simulink model "sm_flex_slider_crank"  (R2020b)
settings: Solver=ode23t  StartTime=0.0  StopTime=1.6  RelTol=1e-3  AbsTol=1e-3
PreLoadFcn:
  | if(~exist('shabanaCrankshaft','var'))
  |   load sliderCrankFEData
  | end
PostLoadFcn:
  | % Enable hard stop
  | hs_on = sm_flex_slider_crank_configure_hardstop(bdroot,'on');
undefined symbols (not defined in the file): beam_wall, beam_width, Extr_Data_Box, shabanaConnectingRod, shabanaCrankshaft, X, Y, Z
libraries: sm_lib x15, nesl_utility x7, sm_flex_body_lib x6, forcesPS_lib x1, fl_lib x1, simulink x1
CloseFcn:
  | try,close(h1_sm_flex_slider_crank),end
  | clear h1_sm_flex_slider_crank
  | try,close(h2_sm_flex_slider_crank),end
  | clear h2_sm_flex_slider_crank
  | try,close(h3_sm_flex_slider_crank),end
  | clear h3_sm_flex_slider_crank
  | try,close(h4_sm_flex_slider_crank),end
  | clear h4_sm_flex_slider_crank
  | 
  | 
  | clear simlog_sm_flex_slider_crank
  | clear logsout_sm_flex_slider_crank
Description:
  | Flexible Body Slider Crank
  | 
  | Copyright 2016-2020 The MathWorks, Inc.
settings Model: Creator=yvanwedd  LastModifiedBy=smiller
settings SolverCC: AutoScaleAbsTol=off
settings DataIOCC: MaxDataPoints=10000  ReturnWorkspaceOutputs=off  SignalLoggingName=logsout_sm_flex_slider_crank
settings DebuggingCC: PregeneratedLibrarySubsystemCodeDiagnostic=none  ArithmeticOperatorsInVariantConditions=warning
settings SFSimCC: SimUseLocalCustomCode=off  CustomCodeUndefinedFunction=UseInterfaceOnly
settings RTWCC: RTWUseLocalCustomCode=off
settings CodeAppCC: StateflowObjectComments=on
settings SimscapeCC: SimscapeNormalizeSystem=off  SimscapeLogType=all  SimscapeLogSimulationStatistics=on  SimscapeLogName=simlog_sm_flex_slider_crank  SimscapeLogLimitData=off  SimscapeLogDataHistory=10000
settings ExplorerConfigSet: InternalSimMechanicsExplorerSettings="<ExplorerConfiguration><canonicalview>default</canonicalview><AnimationSetting><BasePlaybackSpeed>1.0</BasePlaybackSpeed><PlaybackSpeedFactor>1.0</PlaybackSpeedFactor></AnimationSetting><TilePanel><TileInfo><Tiles Columns=\"1\" Count=\"1\" Rows=\"1\"><Column Left=\"2\" Weight=\"1\"/><Column Left=\"599\"/><Row Top=\"2\" Weight=\"1\"/><Row Top=\"397\"/><Tile Height=\"1\" Width=\"1\" X=\"0\" Y=\"0\"/></Tiles></TileInfo><SceneInfo><SceneViewer><BGColor><R>1</R><G>1</G><B>1</B></BGColor><Camera><DoPerspective>off</DoPerspective><Position><X>0.55203353364576724</X><Y>-0.22217409389501411</Y><Z>-0.85738767532460369</Z></Position><Center><X>0.16632771730262594</X><Y>-0.060781097290667566</Y><Z>0.051008341777047675</Z></Center><Up><X>-0.042698376474489097</X><Y>-0.98664868389108351</Y><Z>0.15716622799582453</Z></Up><ViewLimDist>1</ViewLimDist><YLim>0.19284836336170352</YLim><XLim>0.29376900947326862</XLim></Camera></SceneViewer></SceneInfo></TilePanel><MechEditorPanel><Cameras/><GfxPanelCameraMap/><VideoCreator><PlaybackSpeedRatio>1.0</PlaybackSpeedRatio><FrameRate>30</FrameRate><VideoFormat>Motion JPEG AVI</VideoFormat><FrameSize>auto</FrameSize></VideoCreator></MechEditorPanel></ExplorerConfiguration>"

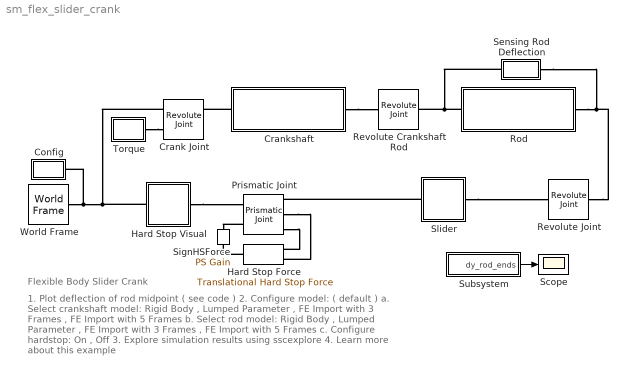
== system sm_flex_slider_crank ==
  note: Flexible Body Slider Crank
  note: 1. Plot deflection of rod midpoint ( see code )
      | 2. Configure model: ( default )
      | a. Select crankshaft model: Rigid Body , Lumped Parameter ,
      | FE Import with 3 Frames , FE Import with 5 Frames
      | b. Select rod model: Rigid Body , Lumped Parameter ,
      | FE Import with 3 Frames , FE Import with 5 Frames
      | c. Configure hardstop: On , Off
      | 3. Explore simulation results using sscexplore
      | 4. Learn more about this example
  Config : Subsystem
  Crank Joint : sm_lib/Joints/Revolute Joint  JointMode=Normal  SenseConstraintForce=off  SenseConstraintForceX=off  SenseConstraintForceY=off  SenseConstraintForceZ=off  SenseConstraintTorque=off  SenseConstraintTorqueX=off  SenseConstraintTorqueY=off  SenseConstraintTorqueZ=off  SenseTotalForce=off  SenseTotalForceX=off  SenseTotalForceY=off  SenseTotalForceZ=off  SenseTotalTorque=off  SenseTotalTorqueX=off  SenseTotalTorqueY=off  SenseTotalTorqueZ=off  CompositeWrenchDir=FollowerOnBase  CompositeWrenchFrame=BaseFrame  EquilibriumPosition=0  EquilibriumPositionUnits=deg  SpringStiffness=0  SpringStiffnessUnits=N*m/deg  DampingCoefficient=0  DampingCoefficientUnits=N*m/(deg/s)  TorqueActuationMode=InputTorque  MotionActuationMode=ComputedMotion  SensePosition=on  SenseVelocity=off  SenseAcceleration=off  SenseTorqueForce=off  SenseLowerLimitTorqueForce=off  SenseUpperLimitTorqueForce=off  LowerLimitSpecify=off  LowerLimitBound=-90  LowerLimitBoundUnits=deg  LowerLimitStiffness=1e4  LowerLimitStiffnessUnits=N*m/deg  LowerLimitDamping=10  LowerLimitDampingUnits=N*m/(deg/s)  LowerLimitTransitionRegionWidth=0.1  LowerLimitTransitionRegionWidthUnits=deg  UpperLimitSpecify=off  UpperLimitBound=90  UpperLimitBoundUnits=deg  UpperLimitStiffness=1e4  UpperLimitStiffnessUnits=N*m/deg  UpperLimitDamping=10  UpperLimitDampingUnits=N*m/(deg/s)  UpperLimitTransitionRegionWidth=0.1  UpperLimitTransitionRegionWidthUnits=deg  PositionTargetSpecify=off  PositionTargetPriority=High  PositionTargetValue=0  PositionTargetValueUnits=deg  VelocityTargetSpecify=off  VelocityTargetPriority=High  VelocityTargetValue=0  VelocityTargetValueUnits=deg/s
  Crankshaft : Subsystem  Variant=on  VariantControlMode=label  VariantControl=Variant1  LabelModeActiveChoice=Rigid_Body
      settings: AttributesFormatString=%<ActiveVariant>
      mask Display:
      | blk = find_system(gcbh, 'SearchDepth', 1, 'Parent', gcb, 'VariantObject', get_param(gcb,'activevariant'));
      | eval(get_param(blk, 'MaskDisplay'));
  Hard Stop Visual : Subsystem
      mask Display:
      | if(evalin('base','hs_on'))
      | patch([1 1 -1 -1],[0.5 1 1 0.5],[0.5 0.5 0.5]);
      | %patch([1 1 -1 -1],[-1 1 1 -1],[0.5 0.5 0.5]);
      | patch([1 1 -1 -1],-[0.5 1 1 0.5],[0.5 0.5 0.5]);
      | else
      | patch([1 1 -1 -1],[-1 1 1 -1],[1 1 1]);
      | end
      | 
      | plot(-2,-2)
      | plot(2,2)
  Hard Stop Force : forcesPS_lib/Mechanical/Translational Hard Stop Force  upper_bnd=0.5 m  lower_bnd=0.3 m  stiff_up=1e6 N/m  stiff_low=1e6 N/m  D_up=150 N/(m/s)  D_low=150 N/(m/s)
      settings: InternalSimscapePortConfiguration="{\"Bottom\":[],\"Left\":[{\"id\":\"v\",\"label\":\"v\",\"type\":\"input\"},{\"id\":\"p\",\"label\":\"p\",\"type\":\"input\"}],\"Right\":[{\"id\":\"f\",\"label\":\"f\",\"type\":\"output\"}],\"Top\":[]}"
  Prismatic Joint : sm_lib/Joints/Prismatic Joint  JointMode=Normal  SenseConstraintForce=off  SenseConstraintForceX=off  SenseConstraintForceY=off  SenseConstraintForceZ=off  SenseConstraintTorque=off  SenseConstraintTorqueX=off  SenseConstraintTorqueY=off  SenseConstraintTorqueZ=off  SenseTotalForce=off  SenseTotalForceX=off  SenseTotalForceY=off  SenseTotalForceZ=off  SenseTotalTorque=off  SenseTotalTorqueX=off  SenseTotalTorqueY=off  SenseTotalTorqueZ=off  CompositeWrenchDir=FollowerOnBase  CompositeWrenchFrame=BaseFrame  EquilibriumPosition=0  EquilibriumPositionUnits=m  SpringStiffness=0  SpringStiffnessUnits=N/m  DampingCoefficient=0  DampingCoefficientUnits=N/(m/s)  TorqueActuationMode=InputTorque  MotionActuationMode=ComputedMotion  SensePosition=on  SenseVelocity=on  SenseAcceleration=off  SenseTorqueForce=off  SenseLowerLimitTorqueForce=off  SenseUpperLimitTorqueForce=off  LowerLimitSpecify=off  LowerLimitBound=-1  LowerLimitBoundUnits=m  LowerLimitStiffness=1e6  LowerLimitStiffnessUnits=N/m  LowerLimitDamping=1e3  LowerLimitDampingUnits=N/(m/s)  LowerLimitTransitionRegionWidth=1e-4  LowerLimitTransitionRegionWidthUnits=m  UpperLimitSpecify=off  UpperLimitBound=1  UpperLimitBoundUnits=m  UpperLimitStiffness=1e6  UpperLimitStiffnessUnits=N/m  UpperLimitDamping=1e3  UpperLimitDampingUnits=N/(m/s)  UpperLimitTransitionRegionWidth=1e-4  UpperLimitTransitionRegionWidthUnits=m  PositionTargetSpecify=on  PositionTargetPriority=High  PositionTargetValue=shabanaCrankshaft.L+shabanaConnectingRod.L  PositionTargetValueUnits=m  VelocityTargetSpecify=on  VelocityTargetPriority=High  VelocityTargetValue=0  VelocityTargetValueUnits=m/s
  Revolute Crankshaft Rod : sm_lib/Joints/Revolute Joint  JointMode=Normal  SenseConstraintForce=off  SenseConstraintForceX=off  SenseConstraintForceY=off  SenseConstraintForceZ=off  SenseConstraintTorque=off  SenseConstraintTorqueX=off  SenseConstraintTorqueY=off  SenseConstraintTorqueZ=off  SenseTotalForce=off  SenseTotalForceX=off  SenseTotalForceY=off  SenseTotalForceZ=off  SenseTotalTorque=off  SenseTotalTorqueX=off  SenseTotalTorqueY=off  SenseTotalTorqueZ=off  CompositeWrenchDir=FollowerOnBase  CompositeWrenchFrame=BaseFrame  EquilibriumPosition=0  EquilibriumPositionUnits=deg  SpringStiffness=0  SpringStiffnessUnits=N*m/deg  DampingCoefficient=0  DampingCoefficientUnits=N*m/(deg/s)  TorqueActuationMode=NoTorque  MotionActuationMode=ComputedMotion  SensePosition=off  SenseVelocity=off  SenseAcceleration=off  SenseTorqueForce=off  SenseLowerLimitTorqueForce=off  SenseUpperLimitTorqueForce=off  LowerLimitSpecify=off  LowerLimitBound=-90  LowerLimitBoundUnits=deg  LowerLimitStiffness=1e4  LowerLimitStiffnessUnits=N*m/deg  LowerLimitDamping=10  LowerLimitDampingUnits=N*m/(deg/s)  LowerLimitTransitionRegionWidth=0.1  LowerLimitTransitionRegionWidthUnits=deg  UpperLimitSpecify=off  UpperLimitBound=90  UpperLimitBoundUnits=deg  UpperLimitStiffness=1e4  UpperLimitStiffnessUnits=N*m/deg  UpperLimitDamping=10  UpperLimitDampingUnits=N*m/(deg/s)  UpperLimitTransitionRegionWidth=0.1  UpperLimitTransitionRegionWidthUnits=deg  PositionTargetSpecify=off  PositionTargetPriority=High  PositionTargetValue=-180  PositionTargetValueUnits=deg  VelocityTargetSpecify=off  VelocityTargetPriority=High  VelocityTargetValue=0  VelocityTargetValueUnits=deg/s
  Revolute Joint : sm_lib/Joints/Revolute Joint  JointMode=Normal  SenseConstraintForce=off  SenseConstraintForceX=off  SenseConstraintForceY=off  SenseConstraintForceZ=off  SenseConstraintTorque=off  SenseConstraintTorqueX=off  SenseConstraintTorqueY=off  SenseConstraintTorqueZ=off  SenseTotalForce=off  SenseTotalForceX=off  SenseTotalForceY=off  SenseTotalForceZ=off  SenseTotalTorque=off  SenseTotalTorqueX=off  SenseTotalTorqueY=off  SenseTotalTorqueZ=off  CompositeWrenchDir=FollowerOnBase  CompositeWrenchFrame=BaseFrame  EquilibriumPosition=0  EquilibriumPositionUnits=deg  SpringStiffness=0  SpringStiffnessUnits=N*m/deg  DampingCoefficient=0  DampingCoefficientUnits=N*m/(deg/s)  TorqueActuationMode=NoTorque  MotionActuationMode=ComputedMotion  SensePosition=off  SenseVelocity=off  SenseAcceleration=off  SenseTorqueForce=off  SenseLowerLimitTorqueForce=off  SenseUpperLimitTorqueForce=off  LowerLimitSpecify=off  LowerLimitBound=-90  LowerLimitBoundUnits=deg  LowerLimitStiffness=1e4  LowerLimitStiffnessUnits=N*m/deg  LowerLimitDamping=10  LowerLimitDampingUnits=N*m/(deg/s)  LowerLimitTransitionRegionWidth=0.1  LowerLimitTransitionRegionWidthUnits=deg  UpperLimitSpecify=off  UpperLimitBound=90  UpperLimitBoundUnits=deg  UpperLimitStiffness=1e4  UpperLimitStiffnessUnits=N*m/deg  UpperLimitDamping=10  UpperLimitDampingUnits=N*m/(deg/s)  UpperLimitTransitionRegionWidth=0.1  UpperLimitTransitionRegionWidthUnits=deg  PositionTargetSpecify=off  PositionTargetPriority=High  PositionTargetValue=0  PositionTargetValueUnits=deg  VelocityTargetSpecify=off  VelocityTargetPriority=High  VelocityTargetValue=0  VelocityTargetValueUnits=deg/s
  Rod : Subsystem  Variant=on  VariantControlMode=label  VariantControl=Variant1  LabelModeActiveChoice=FE_Import_5Frames
      settings: AttributesFormatString=%<ActiveVariant>
      mask Display:
      | blk = find_system(gcbh, 'SearchDepth', 1, 'Parent', gcb, 'VariantObject', get_param(gcb,'activevariant'));
      | eval(get_param(blk, 'MaskDisplay'));
  Scope : Scope
  Sensing Rod Deflection : Subsystem
  SignHSForce : fl_lib/Physical Signals/Functions/PS Gain  Tag=on  gain=-hs_on
      settings: AttributesFormatString=%<Tag>
  Slider : Subsystem
      mask Display:
      | patch([1 1 -1 -1],[-1 1 1 -1],[0.5 0.5 0.5]);
      | plot(-2.5,-2.5)
      | plot(2.5,2.5)
  Subsystem : Subsystem
  Torque : Subsystem
      mask DialogControl Control2 Prompt: No Parameters
  World Frame : sm_lib/Frames and Transforms/World Frame
  wires:
  Subsystem/1(dy_rod_ends) -> Scope/1
  connections:
  Torque/RConn1 -- Crank Joint/LConn2
  Prismatic Joint/RConn2 -- Hard Stop Force/LConn2
  Prismatic Joint/RConn3 -- Hard Stop Force/LConn1
  Prismatic Joint/LConn2 -- SignHSForce/RConn1
  Crankshaft/LConn1 -- Crank Joint/RConn1
  Crankshaft/RConn1 -- Revolute Crankshaft Rod/LConn1
  Rod/LConn1 -- Sensing Rod Deflection/LConn1 -- Revolute Crankshaft Rod/RConn1
  Hard Stop Force/RConn1 -- SignHSForce/LConn1
  Revolute Joint/RConn1 -- Sensing Rod Deflection/RConn1 -- Rod/RConn1
  World Frame/RConn1 -- Hard Stop Visual/RConn1 -- Crank Joint/LConn1 -- Config/RConn1
  Hard Stop Visual/LConn1 -- Prismatic Joint/LConn1
  Slider/LConn1 -- Prismatic Joint/RConn1
  Slider/RConn1 -- Revolute Joint/LConn1

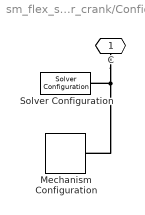
== system sm_flex_slider_crank/Config ==
  Mechanism Configuration : sm_lib/Utilities/Mechanism Configuration  UniformGravity=None  GravityVector=[0 0 -9.80665]  GravityVectorUnits=m/s^2  GravityUnits=m/s^2  LinearizationDelta=0.001  JointModeTransitionNonlinearIterations=2
  Solver Configuration : nesl_utility/Solver Configuration  PhysicalDomain=network_engine_domain  SubClassName=solver  LeftPortType=input  RightPortType=generic  Tones=[]  Harmonics=[]  SimulateNoise=off  Profile=off  UseLocalSampling=off  EnableSwitchedLinearOptims=on  FrequencyDomain=off  UseCCode=off  RelTol=0.001  AbsTol=1e-06  MinStep=1e-09  ToWorkspace=off  RevertToSquareIcSolve=off  NumHomotopyIterations=100  PhasorMode=off  PhasorModeNumHarmonics=1  DoDC=off  ResidualTolerance=1e-09  UseLocalSolver=off  LocalSolverChoice=NE_BACKWARD_EULER_ADVANCER  LocalSolverSampleTime=0.001  DoFixedCost=off  MaxNonlinIter=3  MaxModeIter=2  ComputeImpulses=off  ImpulseIterations=2  LinearAlgebra=Sparse  EquationFormulation=NE_TIME_EF  DelaysMemoryBudget=1024  AutomaticFiltering=on  FilteringTimeConstant=0.001  PartitionStorageMethod=AS_NEEDED  PartitionMemoryBudget=1024  PartitionMethod=FAST
  C : PMIOPort  Side=Right
  connections:
  Mechanism Configuration/RConn1 -- C/RConn1 -- Solver Configuration/RConn1

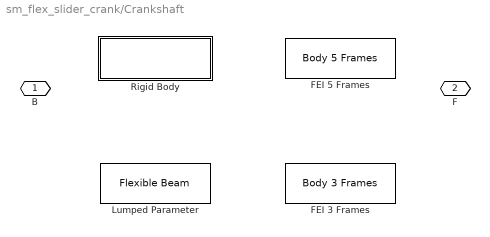
== system sm_flex_slider_crank/Crankshaft ==
  FEI 3 Frames : sm_flex_body_lib/FE Import/Bodies/Body 3 Frames  VariantControl=FE_Import_3Frames  popup_massdistr=Per Interface Frame  mass=shabanaCrankshaft.iner.mass  com=shabanaCrankshaft.iner.com  moi=shabanaCrankshaft.iner.moi  poi=shabanaCrankshaft.iner.poi  splitBodyProps=shabanaCrankshaft.splitBodyProps(2).props  smallInertiaDim=1e-2  smallInertiaMass=1e-4  rigid_body_filename='ShabanaCrankshaft.stl'  rigid_body_color=[0.5 0.5 0.5]  rigid_body_opacity=0  intf_body_color=[0.2 0.4 0.6]  intf_body_opacity=1  intf_graphic_color=[0.1 0.1 0.6]  intf_graphic_opacity=0  rigidBodyFrame=2  T=shabanaCrankshaft.models(5).T  numframes=3  K=shabanaCrankshaft.models(5).K  M=shabanaCrankshaft.models(5).M  ksi=0.05  dofIdxMap=shabanaCrankshaft.models(5).dofIdxMap  tau=1e-7  H=shabanaCrankshaft.models(5).H  sensedFeaDofs_UI=[]  numDynModes=20
      settings: AttributesFormatString=|
      | Mass: %<popup_massdistr>
      | Interface Frames: %<numframes>
      | Rigid Frame: %<rigidBodyFrame>
      | # Dynamic Modes: %<numDynModes>
  FEI 5 Frames : sm_flex_body_lib/FE Import/Bodies/Body 5 Frames  VariantControl=FE_Import_5Frames  popup_massdistr=Single  mass=shabanaCrankshaft.iner.mass  com=shabanaCrankshaft.iner.com  moi=shabanaCrankshaft.iner.moi  poi=shabanaCrankshaft.iner.poi  splitBodyProps=shabanaCrankshaft.splitBodyProps(3).props  smallInertiaDim=1e-2  smallInertiaMass=1e-4  rigid_body_filename='ShabanaCrankshaft.stl'  rigid_body_color=[0.5 0.5 0.5]  rigid_body_opacity=1  intf_body_color=[0.2 0.4 0.6]  intf_body_opacity=0  intf_graphic_color=[0.1 0.1 0.6]  intf_graphic_opacity=0  rigidBodyFrame=3  T=shabanaCrankshaft.models(7).T  numframes=5  K=shabanaCrankshaft.models(7).K  M=shabanaCrankshaft.models(7).M  ksi=0.05  dofIdxMap=shabanaCrankshaft.models(7).dofIdxMap  tau=1e-7  H=shabanaCrankshaft.models(7).H  sensedFeaDofs_UI=[]  numDynModes=20
      settings: AttributesFormatString=|
      | Mass: %<popup_massdistr>
      | Interface Frames: %<numframes>
      | Rigid Frame: %<rigidBodyFrame>
      | # Dynamic Modes: %<numDynModes>
  Lumped Parameter : sm_flex_body_lib/Lumped Parameter/Bodies/Flexible Beam  Tag=PublishSubsystem  VariantControl=Lumped_Parameter  popup_material=Custom  rho_cust=shabanaCrankshaft.mat.rho  youngsM_cust=shabanaCrankshaft.mat.E  shearM_cust=shabanaCrankshaft.mat.G  edf_beam=3.38e-05  sdf_beam=3.38e-05  checkbox_internalvalues=off  popup_xc=Hollow Rectangle  beam_width=shabanaCrankshaft.cs.b  beam_width_in=0  beam_height=shabanaCrankshaft.cs.a  beam_height_in=0  circle_diameter=0.015  circle_diameter_in=0  custom_ixx=2.6121e-003  custom_iyy=2.6121e-003  custom_ip=5.2242e-003  custom_j=5.2242e-003  extrusion_data_custom=[0.015 0.005;-0.015 0.005;-0.015 -0.005;0.015 -0.005]/2  beam_length=shabanaCrankshaft.L  elem_length=0.0152  numelem=10  extrusion_data=Extr_Data_Box(beam_width,beam_width-2*beam_wall,beam_width,beam_width-2*beam_wall)  beam_color=[0 0.4 0.6]  beam_opacity=1  radio_flextype=Rotation: Z
      settings: AttributesFormatString=|
      | No of Elem: 10
      | Rotation: Z
  Rigid Body : Subsystem  VariantControl=Rigid_Body
      mask Display: image('sm_flex_body_lib_rigidbody_IMAGE.png')
  " B " : PMIOPort  Side=Left
  " F " : PMIOPort  Port=2  Side=Right

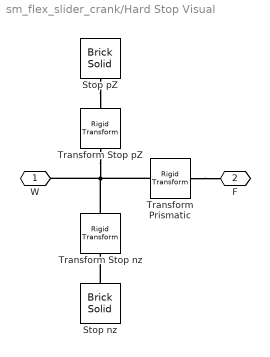
== system sm_flex_slider_crank/Hard Stop Visual ==
  Stop nz : sm_lib/Body Elements/Brick Solid  GraphicAmbientColor=[0.15 0.15 0.15 1.0]  BasedOnType=Density  BrickDimensions=[0.04 0.02 0.02]  BrickDimensionUnits=m  CenterOfMass=[0 0 0]  CenterOfMassUnits=m  GraphicDiffuseColor=[0.5 0.5 0.5]  Density=1000  DensityUnits=kg/m^3  DoExposeReferenceFrame=off  GraphicEmissiveColor=[0.0 0.0 0.0 1.0]  ExportEntireGeometry=off  SerializedFrames=<Frames><Frame><Id>Frame1</Id><Value><Name>F</Name><Origin><Source>GeometricFeature</Source><FeatureName>-z +x curve</FeatureName></Origin><PrimaryAxis><DefinedDirection>+Z</DefinedDirection><Source>ReferenceFrame</Source><SourceDirection>+Z</SourceDirection><FeatureName></FeatureName></PrimaryAxis><SecondaryAxis><DefinedDirection>+Y</DefinedDirection><Source>ReferenceFrame</Source><SourceDirection>+Y</SourceDirection><FeatureName></FeatureName></SecondaryAxis></Value></Frame></Frames>  MarkerShape=Sphere  MarkerSize=10  GraphicType=FromGeometry  InertiaType=PointMass  Mass=0  MassUnits=kg  MomentsOfInertia=[1 1 1]  MomentsOfInertiaUnits=kg*m^2  GraphicOpacity=hs_on*0.5  ProductsOfInertia=[1 1 1]  ProductsOfInertiaUnits=kg*m^2  GraphicShininess=75  GraphicSpecularColor=[0.5 0.5 0.5 1.0]  GraphicVisPropType=SimpleVisualProperties
  Stop pZ : sm_lib/Body Elements/Brick Solid  GraphicAmbientColor=[0.15 0.15 0.15 1.0]  BasedOnType=Density  BrickDimensions=[0.04 0.02 0.02]  BrickDimensionUnits=m  CenterOfMass=[0 0 0]  CenterOfMassUnits=m  GraphicDiffuseColor=[0.5 0.5 0.5]  Density=1000  DensityUnits=kg/m^3  DoExposeReferenceFrame=off  GraphicEmissiveColor=[0.0 0.0 0.0 1.0]  ExportEntireGeometry=off  SerializedFrames=<Frames><Frame><Id>Frame1</Id><Value><Name>F</Name><Origin><Source>GeometricFeature</Source><FeatureName>+z +x curve</FeatureName></Origin><PrimaryAxis><DefinedDirection>+Z</DefinedDirection><Source>ReferenceFrame</Source><SourceDirection>+Z</SourceDirection><FeatureName></FeatureName></PrimaryAxis><SecondaryAxis><DefinedDirection>+Y</DefinedDirection><Source>ReferenceFrame</Source><SourceDirection>+Y</SourceDirection><FeatureName></FeatureName></SecondaryAxis></Value></Frame></Frames>  MarkerShape=Sphere  MarkerSize=10  GraphicType=FromGeometry  InertiaType=PointMass  Mass=0  MassUnits=kg  MomentsOfInertia=[1 1 1]  MomentsOfInertiaUnits=kg*m^2  GraphicOpacity=hs_on*0.5  ProductsOfInertia=[1 1 1]  ProductsOfInertiaUnits=kg*m^2  GraphicShininess=75  GraphicSpecularColor=[0.5 0.5 0.5 1.0]  GraphicVisPropType=SimpleVisualProperties
  Transform Prismatic : sm_lib/Frames and Transforms/Rigid Transform  TranslationMethod=None  TranslationStandardOffset=0  TranslationLengthUnit=m  TranslationStandardAxis=+Z  TranslationCartesianOffset=[0 0 0]  TranslationROffset=0  TranslationROffsetUnits=m  TranslationZOffset=0  TranslationZOffsetUnits=m  TranslationThetaOffset=0  TranslationThetaOffsetUnits=deg  RotationMethod=StandardAxis  RotationAngleUnits=deg  RotationStandardAxis=+Y  RotationAngle=90  RotationArbitraryAxis=[0 0 1]  FollAlignAxisA=+X  BaseAlignAxisA=+Y  FollAlignAxisB=+Y  BaseAlignAxisB=+Z  RotationSequenceAxes=FollowerAxes  RotationSequence=XYX  RotationSequenceAngles=[0 0 0]  RotationSequenceAnglesUnits=deg  RotationMatrix=[1 0 0; 0 1 0; 0 0 1]
  Transform Stop nz : sm_lib/Frames and Transforms/Rigid Transform  TranslationMethod=Cartesian  TranslationStandardOffset=0  TranslationLengthUnit=m  TranslationStandardAxis=-Z  TranslationCartesianOffset=[0.3 0 shabanaConnectingRod.cs.a]  TranslationROffset=0  TranslationROffsetUnits=m  TranslationZOffset=0  TranslationZOffsetUnits=m  TranslationThetaOffset=0  TranslationThetaOffsetUnits=deg  RotationMethod=None  RotationAngleUnits=deg  RotationStandardAxis=+Y  RotationAngle=90  RotationArbitraryAxis=[0 0 1]  FollAlignAxisA=+X  BaseAlignAxisA=+Y  FollAlignAxisB=+Y  BaseAlignAxisB=+Z  RotationSequenceAxes=FollowerAxes  RotationSequence=XYX  RotationSequenceAngles=[0 0 0]  RotationSequenceAnglesUnits=deg  RotationMatrix=[1 0 0; 0 1 0; 0 0 1]
  Transform Stop pZ : sm_lib/Frames and Transforms/Rigid Transform  TranslationMethod=Cartesian  TranslationStandardOffset=0  TranslationLengthUnit=m  TranslationStandardAxis=-Z  TranslationCartesianOffset=[0.3 0 -shabanaConnectingRod.cs.a]  TranslationROffset=0  TranslationROffsetUnits=m  TranslationZOffset=0  TranslationZOffsetUnits=m  TranslationThetaOffset=0  TranslationThetaOffsetUnits=deg  RotationMethod=None  RotationAngleUnits=deg  RotationStandardAxis=+Y  RotationAngle=90  RotationArbitraryAxis=[0 0 1]  FollAlignAxisA=+X  BaseAlignAxisA=+Y  FollAlignAxisB=+Y  BaseAlignAxisB=+Z  RotationSequenceAxes=FollowerAxes  RotationSequence=XYX  RotationSequenceAngles=[0 0 0]  RotationSequenceAnglesUnits=deg  RotationMatrix=[1 0 0; 0 1 0; 0 0 1]
  W : PMIOPort  Side=Right
  F : PMIOPort  Port=2  Side=Left
  connections:
  Transform Prismatic/LConn1 -- Transform Stop nz/LConn1 -- Transform Stop pZ/LConn1 -- W/RConn1
  Transform Prismatic/RConn1 -- F/RConn1
  Stop pZ/LConn1 -- Transform Stop pZ/RConn1
  Stop nz/LConn1 -- Transform Stop nz/RConn1

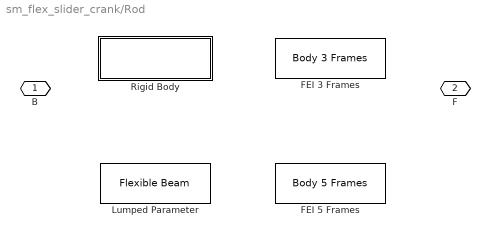
== system sm_flex_slider_crank/Rod ==
  FEI 3 Frames : sm_flex_body_lib/FE Import/Bodies/Body 3 Frames  VariantControl=FE_Import_3Frames  popup_massdistr=Per Interface Frame  mass=shabanaConnectingRod.iner.mass  com=shabanaConnectingRod.iner.com  moi=shabanaConnectingRod.iner.moi  poi=shabanaConnectingRod.iner.poi  splitBodyProps=shabanaConnectingRod.splitBodyProps(2).props  smallInertiaDim=1e-3  smallInertiaMass=1e-6  rigid_body_filename='ShabanaConnectingRod.step'  rigid_body_color=[0.5 0.5 0.5]  rigid_body_opacity=0  intf_body_color=[0.2 0.4 0.6]  intf_body_opacity=1  intf_graphic_color=[0.1 0.1 0.6]  intf_graphic_opacity=0  rigidBodyFrame=2  T=shabanaConnectingRod.models(5).T  numframes=3  K=shabanaConnectingRod.models(5).K  M=shabanaConnectingRod.models(5).M  ksi=0.05  dofIdxMap=shabanaConnectingRod.models(5).dofIdxMap  tau=1e-7  H=shabanaConnectingRod.models(5).H  sensedFeaDofs_UI=[]  numDynModes=20
      settings: AttributesFormatString=|
      | Mass: %<popup_massdistr>
      | Interface Frames: %<numframes>
      | Rigid Frame: %<rigidBodyFrame>
      | # Dynamic Modes: %<numDynModes>
  FEI 5 Frames : sm_flex_body_lib/FE Import/Bodies/Body 5 Frames  VariantControl=FE_Import_5Frames  popup_massdistr=Per Interface Frame  mass=shabanaConnectingRod.iner.mass  com=shabanaConnectingRod.iner.com  moi=shabanaConnectingRod.iner.moi  poi=shabanaConnectingRod.iner.poi  splitBodyProps=shabanaConnectingRod.splitBodyProps(3).props  smallInertiaDim=1e-3  smallInertiaMass=1e-6  rigid_body_filename='ShabanaConnectingRod.stl'  rigid_body_color=[0.5 0.5 0.5]  rigid_body_opacity=0  intf_body_color=[0.2 0.4 0.6]  intf_body_opacity=1  intf_graphic_color=[0.1 0.1 0.6]  intf_graphic_opacity=0  rigidBodyFrame=3  T=shabanaConnectingRod.models(7).T  numframes=5  K=shabanaConnectingRod.models(7).K  M=shabanaConnectingRod.models(7).M  ksi=0.05  dofIdxMap=shabanaConnectingRod.models(7).dofIdxMap  tau=1e-7  H=shabanaConnectingRod.models(7).H  sensedFeaDofs_UI=[]  numDynModes=20
      settings: AttributesFormatString=|
      | Mass: %<popup_massdistr>
      | Interface Frames: %<numframes>
      | Rigid Frame: %<rigidBodyFrame>
      | # Dynamic Modes: %<numDynModes>
  Lumped Parameter : sm_flex_body_lib/Lumped Parameter/Bodies/Flexible Beam  Tag=PublishSubsystem  VariantControl=Lumped_Parameter  popup_material=Custom  rho_cust=shabanaConnectingRod.mat.rho  youngsM_cust=shabanaConnectingRod.mat.E  shearM_cust=shabanaConnectingRod.mat.G  edf_beam=6.03e-04  sdf_beam=6.03e-04  checkbox_internalvalues=off  popup_xc=Hollow Rectangle  beam_width=shabanaConnectingRod.cs.b  beam_width_in=0  beam_height=shabanaConnectingRod.cs.a  beam_height_in=0  circle_diameter=0.015  circle_diameter_in=0  custom_ixx=2.6121e-003  custom_iyy=2.6121e-003  custom_ip=5.2242e-003  custom_j=5.2242e-003  extrusion_data_custom=[0.015 0.005;-0.015 0.005;-0.015 -0.005;0.015 -0.005]/2  beam_length=shabanaConnectingRod.L  elem_length=0.0152  numelem=20  extrusion_data=Extr_Data_Box(beam_width,beam_width-2*beam_wall,beam_width,beam_width-2*beam_wall)  beam_color=[0.6 0.4 0]  beam_opacity=1  radio_flextype=Rotation: Z
      settings: AttributesFormatString=|
      | No of Elem: 20
      | Rotation: Z
  Rigid Body : Subsystem  VariantControl=Rigid_Body
      mask Display: image('sm_flex_body_lib_rigidbody_IMAGE.png')
  " B " : PMIOPort  Side=Left
  " F " : PMIOPort  Port=2  Side=Right

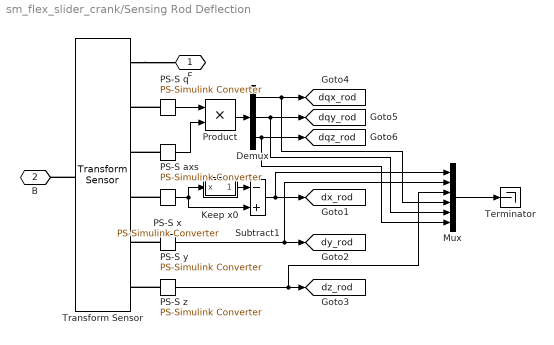
== system sm_flex_slider_crank/Sensing Rod Deflection ==
  Demux : Demux  Outputs=3
  Keep x0 : Subsystem
  Mux : Mux  Inputs=6
  PS-S axs : nesl_utility/PS-Simulink Converter  PhysicalDomain=network_engine_domain  SubClassName=ps_output  LeftPortType=input  RightPortType=output  PseudoPeriodic=off  Frequencies=[]  Unit=1  AffineConversion=off
  PS-S q : nesl_utility/PS-Simulink Converter  PhysicalDomain=network_engine_domain  SubClassName=ps_output  LeftPortType=input  RightPortType=output  PseudoPeriodic=off  Frequencies=[]  Unit=rad  AffineConversion=off
  PS-S x : nesl_utility/PS-Simulink Converter  PhysicalDomain=network_engine_domain  SubClassName=ps_output  LeftPortType=input  RightPortType=output  PseudoPeriodic=off  Frequencies=[]  Unit=m  AffineConversion=off
  PS-S y : nesl_utility/PS-Simulink Converter  PhysicalDomain=network_engine_domain  SubClassName=ps_output  LeftPortType=input  RightPortType=output  PseudoPeriodic=off  Frequencies=[]  Unit=m  AffineConversion=off
  PS-S z : nesl_utility/PS-Simulink Converter  PhysicalDomain=network_engine_domain  SubClassName=ps_output  LeftPortType=input  RightPortType=output  PseudoPeriodic=off  Frequencies=[]  Unit=m  AffineConversion=off
  Product : Product
  Subtract1 : Sum  Inputs=-+
  Terminator : Terminator
  Transform Sensor : sm_lib/Frames and Transforms/Transform Sensor  MeasurementFrame=Base  SenseAngle=on  SenseAxis=on  SenseAngle1=off  SenseAngle2=off  SenseAngle3=off  SenseQ=off  SenseR=off  SenseOmegaX=off  SenseOmegaY=off  SenseOmegaZ=off  SenseOmega1=off  SenseOmega2=off  SenseOmega3=off  SenseQDot=off  SenseRDot=off  SenseAlphaX=off  SenseAlphaY=off  SenseAlphaZ=off  SenseAlpha1=off  SenseAlpha2=off  SenseAlpha3=off  SenseQDDot=off  SenseRDDot=off  SenseX=on  SenseY=on  SenseZ=on  SenseRad=off  SenseAzim=off  SenseDist=off  SenseInc=off  SenseXDot=off  SenseYDot=off  SenseZDot=off  SenseRadDot=off  SenseAzimDot=off  SenseDistDot=off  SenseIncDot=off  SenseXDDot=off  SenseYDDot=off  SenseZDDot=off  SenseRadDDot=off  SenseAzimDDot=off  SenseDistDDot=off  SenseIncDDot=off
  F : PMIOPort  Side=Right
  B : PMIOPort  Port=2  Side=Left
  tag scope: dqx_rod=global, dqy_rod=global, dqz_rod=global, dx_rod=global, dy_rod=global, dz_rod=global
  wires:
  PS-S axs/1 -> Product/2
  PS-S q/1 -> Product/1
  PS-S z/1 -> Mux/3, [dz_rod]
  PS-S y/1 -> Mux/2, [dy_rod]
  Mux/1 -> Terminator/1
  Product/1 -> Demux/1
  Demux/1 -> Mux/4, [dqx_rod]
  Demux/2 -> [dqy_rod], Mux/5
  Demux/3 -> Mux/6, [dqz_rod]
  Subtract1/1 -> [dx_rod], Mux/1
  PS-S x/1 -> Keep x0/1(x), Subtract1/2
  Keep x0/1(x0) -> Subtract1/1
  connections:
  PS-S y/LConn1 -- Transform Sensor/RConn5
  PS-S axs/LConn1 -- Transform Sensor/RConn3
  Transform Sensor/RConn1 -- F/RConn1
  PS-S q/LConn1 -- Transform Sensor/RConn2
  Transform Sensor/LConn1 -- B/RConn1
  PS-S x/LConn1 -- Transform Sensor/RConn4
  PS-S z/LConn1 -- Transform Sensor/RConn6

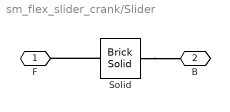
== system sm_flex_slider_crank/Slider ==
  Solid : sm_lib/Body Elements/Brick Solid  GraphicAmbientColor=[0.15 0.15 0.15 1.0]  BasedOnType=Density  BrickDimensions=[0.04 0.02 0.04]  BrickDimensionUnits=m  CenterOfMass=[0 0 0]  CenterOfMassUnits=m  GraphicDiffuseColor=[0.5 0.5 0.5]  Density=1000  DensityUnits=kg/m^3  DoExposeReferenceFrame=off  GraphicEmissiveColor=[0.0 0.0 0.0 1.0]  ExportEntireGeometry=off  SerializedFrames=<Frames><Frame><Id>Frame1</Id><Value><Name>F</Name><Origin><Source>GeometricFeature</Source><FeatureName>-x surface</FeatureName></Origin><PrimaryAxis><DefinedDirection>+Z</DefinedDirection><Source>ReferenceFrame</Source><SourceDirection>+X</SourceDirection><FeatureName></FeatureName></PrimaryAxis><SecondaryAxis><DefinedDirection>+Y</DefinedDirection><Source>ReferenceFrame</Source><SourceDirection>+Y</SourceDirection><FeatureName></FeatureName></SecondaryAxis></Value></Frame><Frame><Id>Frame2</Id><Value><Name>B</Name><Origin><Source>GeometricFeature</Source><FeatureName>-x surface</FeatureName></Origin><PrimaryAxis><DefinedDirection>+Z</DefinedDirection><Source>ReferenceFrame</Source><SourceDirection>+Z</SourceDirection><FeatureName></FeatureName></PrimaryAxis><SecondaryAxis><DefinedDirection>+X</DefinedDirection><Source>ReferenceFrame</Source><SourceDirection>+X</SourceDirection><FeatureName></FeatureName></SecondaryAxis></Value></Frame></Frames>  MarkerShape=Sphere  MarkerSize=10  GraphicType=FromGeometry  InertiaType=PointMass  Mass=0  MassUnits=kg  MomentsOfInertia=[1 1 1]  MomentsOfInertiaUnits=kg*m^2  GraphicOpacity=0.5  ProductsOfInertia=[1 1 1]  ProductsOfInertiaUnits=kg*m^2  GraphicShininess=75  GraphicSpecularColor=[0.5 0.5 0.5 1.0]  GraphicVisPropType=SimpleVisualProperties
  F : PMIOPort  Side=Left
  B : PMIOPort  Port=2  Side=Right
  connections:
  Solid/RConn1 -- B/RConn1
  Solid/LConn1 -- F/RConn1

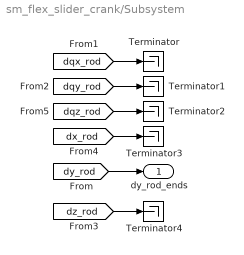
== system sm_flex_slider_crank/Subsystem ==
  Terminator{,1..4} (5 alike) : Terminator
  dy_rod_ends : Outport  VectorParamsAs1DForOutWhenUnconnected=off
  wires:
  [dy_rod] -> dy_rod_ends/1
  [dqx_rod] -> Terminator/1
  [dqy_rod] -> Terminator1/1
  [dqz_rod] -> Terminator2/1
  [dx_rod] -> Terminator3/1
  [dz_rod] -> Terminator4/1

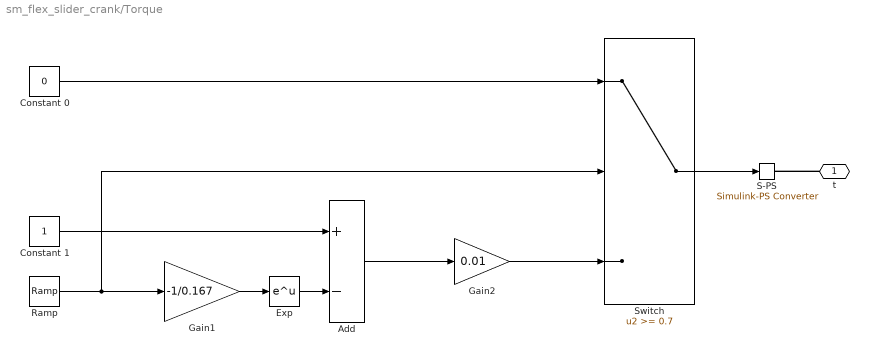
== system sm_flex_slider_crank/Torque ==
  Add : Sum  Inputs=+-
  Constant 0 : Constant  Value=0
  Constant 1 : Constant
  Exp : Math  SignedPower=on  SaturateOnIntegerOverflow=on
  Gain1 : Gain  Gain=-1/0.167
  Gain2 : Gain  Gain=0.01
  Ramp : simulink/Sources/Ramp  slope=1  start=0  InitialOutput=0
  S-PS : nesl_utility/Simulink-PS Converter  PhysicalDomain=network_engine_domain  SubClassName=ps_input  LeftPortType=input  RightPortType=output  PseudoPeriodic=off  Frequencies=[]  NoiseDistribution=none  NoiseParameters=[]  Unit=N*m  AffineConversion=off  FilteringAndDerivatives=zero  SimscapeFilterOrder=1  InputFilterTimeConstant=0.001  UdotUserProvided=1
  Switch : Switch  Threshold=0.7
  t : PMIOPort  Side=Right
  wires:
  Switch/1 -> S-PS/1
  Gain2/1 -> Switch/3
  Constant 0/1 -> Switch/1
  Exp/1 -> Add/2
  Constant 1/1 -> Add/1
  Add/1 -> Gain2/1
  Gain1/1 -> Exp/1
  Ramp/1 -> Gain1/1, Switch/2
  connections:
  t/RConn1 -- S-PS/RConn1

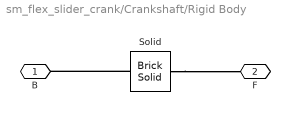
== system sm_flex_slider_crank/Crankshaft/Rigid Body ==
  Solid : sm_lib/Body Elements/Brick Solid  GraphicAmbientColor=[0.15 0.15 0.15 1.0]  BasedOnType=Density  BrickDimensions=[shabanaCrankshaft.L shabanaCrankshaft.cs.b shabanaCrankshaft.cs.a]  BrickDimensionUnits=m  CenterOfMass=[0 0 0]  CenterOfMassUnits=m  GraphicDiffuseColor=[0.5 0.5 0.5]  Density=1000  DensityUnits=kg/m^3  DoExposeReferenceFrame=off  GraphicEmissiveColor=[0.0 0.0 0.0 1.0]  ExportEntireGeometry=off  SerializedFrames=<Frames><Frame><Id>Frame1</Id><Value><Name>B</Name><Origin><Source>GeometricFeature</Source><FeatureName>-x surface</FeatureName></Origin><PrimaryAxis><DefinedDirection>+Z</DefinedDirection><Source>ReferenceFrame</Source><SourceDirection>+Z</SourceDirection><FeatureName></FeatureName></PrimaryAxis><SecondaryAxis><DefinedDirection>+X</DefinedDirection><Source>ReferenceFrame</Source><SourceDirection>+X</SourceDirection><FeatureName></FeatureName></SecondaryAxis></Value></Frame><Frame><Id>Frame2</Id><Value><Name>F</Name><Origin><Source>GeometricFeature</Source><FeatureName>+x surface</FeatureName></Origin><PrimaryAxis><DefinedDirection>+Z</DefinedDirection><Source>ReferenceFrame</Source><SourceDirection>+Z</SourceDirection><FeatureName></FeatureName></PrimaryAxis><SecondaryAxis><DefinedDirection>+X</DefinedDirection><Source>ReferenceFrame</Source><SourceDirection>+X</SourceDirection><FeatureName></FeatureName></SecondaryAxis></Value></Frame></Frames>  MarkerShape=Sphere  MarkerSize=10  GraphicType=FromGeometry  InertiaType=Custom  Mass=shabanaCrankshaft.iner.mass  MassUnits=kg  MomentsOfInertia=shabanaCrankshaft.iner.moi  MomentsOfInertiaUnits=kg*m^2  GraphicOpacity=1.0  ProductsOfInertia=shabanaCrankshaft.iner.poi  ProductsOfInertiaUnits=kg*m^2  GraphicShininess=75  GraphicSpecularColor=[0.5 0.5 0.5 1.0]  GraphicVisPropType=SimpleVisualProperties
  " B " : PMIOPort  Side=Left
  " F " : PMIOPort  Port=2  Side=Right
  connections:
  Solid/LConn1 -- " B "/RConn1
  Solid/RConn1 -- " F "/RConn1

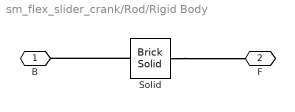
== system sm_flex_slider_crank/Rod/Rigid Body ==
  Solid : sm_lib/Body Elements/Brick Solid  GraphicAmbientColor=[0.15 0.15 0.15 1.0]  BasedOnType=Density  BrickDimensions=[shabanaConnectingRod.L shabanaConnectingRod.cs.b shabanaConnectingRod.cs.a]  BrickDimensionUnits=m  CenterOfMass=[0 0 0]  CenterOfMassUnits=m  GraphicDiffuseColor=[0.5 0.5 0.5]  Density=1000  DensityUnits=kg/m^3  DoExposeReferenceFrame=off  GraphicEmissiveColor=[0.0 0.0 0.0 1.0]  ExportEntireGeometry=off  SerializedFrames=<Frames><Frame><Id>Frame1</Id><Value><Name>B</Name><Origin><Source>GeometricFeature</Source><FeatureName>-x surface</FeatureName></Origin><PrimaryAxis><DefinedDirection>+Z</DefinedDirection><Source>ReferenceFrame</Source><SourceDirection>+Z</SourceDirection><FeatureName></FeatureName></PrimaryAxis><SecondaryAxis><DefinedDirection>+X</DefinedDirection><Source>ReferenceFrame</Source><SourceDirection>+X</SourceDirection><FeatureName></FeatureName></SecondaryAxis></Value></Frame><Frame><Id>Frame2</Id><Value><Name>F</Name><Origin><Source>GeometricFeature</Source><FeatureName>+x surface</FeatureName></Origin><PrimaryAxis><DefinedDirection>+Z</DefinedDirection><Source>ReferenceFrame</Source><SourceDirection>+Z</SourceDirection><FeatureName></FeatureName></PrimaryAxis><SecondaryAxis><DefinedDirection>+X</DefinedDirection><Source>ReferenceFrame</Source><SourceDirection>+X</SourceDirection><FeatureName></FeatureName></SecondaryAxis></Value></Frame></Frames>  MarkerShape=Sphere  MarkerSize=10  GraphicType=FromGeometry  InertiaType=Custom  Mass=shabanaConnectingRod.iner.mass  MassUnits=kg  MomentsOfInertia=shabanaConnectingRod.iner.moi  MomentsOfInertiaUnits=kg*m^2  GraphicOpacity=1.0  ProductsOfInertia=shabanaConnectingRod.iner.poi  ProductsOfInertiaUnits=kg*m^2  GraphicShininess=75  GraphicSpecularColor=[0.5 0.5 0.5 1.0]  GraphicVisPropType=SimpleVisualProperties
  " B " : PMIOPort  Side=Left
  " F " : PMIOPort  Port=2  Side=Right
  connections:
  Solid/LConn1 -- " B "/RConn1
  Solid/RConn1 -- " F "/RConn1

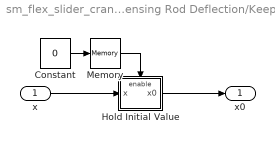
== system sm_flex_slider_crank/Sensing Rod Deflection/Keep x0 ==
  x : Inport
  Constant : Constant  Value=0
  Hold Initial Value : Subsystem
  Memory : Memory  InitialCondition=1
  x0 : Outport  VectorParamsAs1DForOutWhenUnconnected=off
  wires:
  Constant/1 -> Memory/1
  Hold Initial Value/1(x0) -> x0/1
  x/1 -> Hold Initial Value/1(x)
  Memory/1 -> Hold Initial Value/Enable

== system sm_flex_slider_crank/Sensing Rod Deflection/Keep x0/Hold Initial Value ==
  x : Inport
  Enable : EnablePort
  x0 : Outport  VectorParamsAs1DForOutWhenUnconnected=off
  wires:
  x/1 -> x0/1
